simulink model "nonlinear_model1"  (R2021b)
settings: Solver=FixedStepAuto  StartTime=0.0  StopTime=RunTime  FixedStep=time_step  RelTol=1e-3
values from neighbouring files (symbols this model uses):
  g1 = (m_1 * c_1_0 + m_2 * l_1) * g    [compare_ourmodel_with_others.m]    (also in step4_0_linearize_operating_point.m = (m1 * c1 + m2 * l1) * g; step6_1_controller_feedback.m = (m1 * c1 + m2 * l1) * g)
  g2 = m_2 * c_2_0 * g    [compare_ourmodel_with_others.m]    (also in step4_0_linearize_operating_point.m = m2 * c2 * g; step6_1_controller_feedback.m = m2 * c2 * g)
  init_theta_1 = pi    (= 3.14159265359)    [compare_ourmodel_with_others.m]    (also in step2_whitebox_beam.m = theta_1(1); step2_whitebox_pend.m)
  init_theta_2 = 0    [compare_ourmodel_with_others.m]    (also in step2_whitebox_beam.m = theta_1(2); step2_whitebox_pend.m = -1.57079632679)
  P1 = m_1 * c_1_0 * c_1_0 + m_2 * l_1 * l_1 + I_1_0    [compare_ourmodel_with_others.m]    (also in step4_0_linearize_operating_point.m = m1 * c1 * c1 + m2 * l1 * l1 + I1; step6_1_controller_feedback.m = m1 * c1 * c1 + m2 * l1 * l1 + I1)
  P2 = m_2 * c_2_0 * c_2_0 + I_2_0    [compare_ourmodel_with_others.m]    (also in step4_0_linearize_operating_point.m = m2 * c2 * c2 + I2; step6_1_controller_feedback.m = m2 * c2 * c2 + I2)
  P3 = m_2 * l_1 * c_2_0    [compare_ourmodel_with_others.m]    (also in step4_0_linearize_operating_point.m = m2 * l1 * c2; step6_1_controller_feedback.m = m2 * l1 * c2)
  params = [9.81, 0.1, 0.1, 0.125, 0.0487, -0.0286, 0.0624, 0.0169, 6.81e-5, 6.9742, 2.89e-05, 46.1069, 0.0308]    [compare_ourmodel_with_others.m]    (also in costfun.m = x; step2_whitebox_pend.m = x; step4_linearized_system.mat = [9.81 0.1 0.1 0.125 0.046955 -0.032 0.04609 0.0088 9.8e-05 6)
settings Model: Creator=97083  LastModifiedBy=97083
settings DataIOCC: ExternalInput=[u]
settings DebuggingCC: UnconnectedInputMsg=none  UnconnectedOutputMsg=none  UnconnectedLineMsg=none  UnderSpecifiedDimensionMsg=warning
settings ModelReferenceCC: EnableRefExpFcnMdlSchedulingChecks=off
settings RTWCC: DLArmComputeVersion=20.02.1

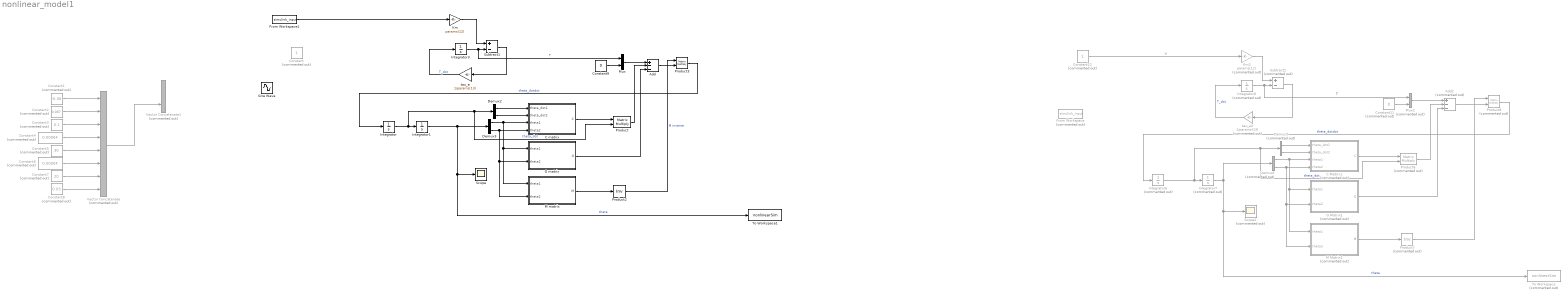
== system nonlinear_model1 ==
  Add : Sum  Inputs=+--
  Add2 : Sum  Commented=on  Inputs=+--
  C Matrix1 : MATLAB Function  Commented=on  TreatAsAtomicUnit=on
  C matrix : MATLAB Function  TreatAsAtomicUnit=on
  Constant : Constant  Commented=on
  Constant1 : Constant  Commented=on  Value=-0.06
  Constant11 : Constant  Commented=on  Value=0
  Constant12 : Constant  Commented=on
  Constant2 : Constant  Commented=on  Value=0.087
  Constant3 : Constant  Commented=on  Value=0.1
  Constant4 : Constant  Commented=on  Value=0.00004
  Constant5 : Constant  Commented=on  Value=30
  Constant6 : Constant  Commented=on  Value=0.00004
  Constant7 : Constant  Commented=on  Value=20
  Constant8 : Constant  Commented=on  Value=0.03
  Constant9 : Constant  Value=0
  Demux2 : Demux  Outputs=2
  Demux3 : Demux  Outputs=2
  Demux5 : Demux  Commented=on  Outputs=2
  Demux6 : Demux  Commented=on  Outputs=2
  From Workspace : FromWorkspace  Commented=on  SampleTime=-1
  From Workspace1 : FromWorkspace  SampleTime=-1
  G Matrix1 : MATLAB Function  Commented=on  TreatAsAtomicUnit=on
  G matrix : MATLAB Function  TreatAsAtomicUnit=on
  Integrator : Integrator
  Integrator1 : Integrator  InitialCondition=[init_theta_1, init_theta_2]
  Integrator3 : Integrator
  Integrator6 : Integrator  Commented=on
  Integrator7 : Integrator  Commented=on  InitialCondition=[init_theta_1, init_theta_2]
  Integrator8 : Integrator  Commented=on
  Km : Gain  Gain=params(12)
  Km2 : Gain  Commented=on  Gain=params(12)
  M Matrix1 : MATLAB Function  Commented=on  TreatAsAtomicUnit=on
  M matrix : MATLAB Function  TreatAsAtomicUnit=on
  Mux : Mux  Inputs=2
  Mux2 : Mux  Commented=on  Inputs=2
  Product : Product  Inputs=**  Multiplication=Matrix(*)
  Product2 : Product  Inputs=/  Multiplication=Matrix(*)
  Product3 : Product  Inputs=**  Multiplication=Matrix(*)
  Product6 : Product  Commented=on  Inputs=**  Multiplication=Matrix(*)
  Product7 : Product  Commented=on  Inputs=/  Multiplication=Matrix(*)
  Product8 : Product  Commented=on  Inputs=**  Multiplication=Matrix(*)
  Scope : Scope
  Scope2 : Scope  Commented=on
  Sine Wave : Sin  Amplitude=4  Frequency=4  SampleTime=0
  Subtract1 : Sum  Inputs=+-
  Subtract2 : Sum  Commented=on  Inputs=+-
  To Workspace : ToWorkspace  Commented=on  VariableName=nonlinearSim  SampleTime=0.001
  To Workspace1 : ToWorkspace  VariableName=nonlinearSim  SampleTime=0.001
  Vector Concatenate : Concatenate  Commented=on  NumInputs=8
  Vector Concatenate1 : Concatenate  Commented=on
  tau_e : Gain  Gain=1/params(13)
  tau_e2 : Gain  Commented=on  Gain=1/params(13)
  wires:
  Constant1/1 -> Vector Concatenate/1
  Constant2/1 -> Vector Concatenate/2
  Constant3/1 -> Vector Concatenate/3
  Constant4/1 -> Vector Concatenate/4
  Constant5/1 -> Vector Concatenate/5
  Constant6/1 -> Vector Concatenate/6
  Constant7/1 -> Vector Concatenate/7
  Constant8/1 -> Vector Concatenate/8
  ? -> Vector Concatenate1/1
  Vector Concatenate/1 -> Vector Concatenate1/2
  G matrix/1(G) -> Add/3
  From Workspace1/1 -> Km/1
  Product/1 -> Add/2
  Subtract1/1 -> tau_e/1
  Add/1 -> Product3/2
  Demux2/1 -> C matrix/1(theta_dot1)
  Constant9/1 -> Mux/2
  Integrator3/1 -> Mux/1, Subtract1/2  "T"
  tau_e/1 -> Integrator3/1  "T_dot"
  Demux3/1 -> M matrix/1(theta1), G matrix/1(theta1), C matrix/3(theta1)
  Product2/1 -> Product3/1  "M inverse"
  Product3/1 -> Integrator/1  "theta_dotdot"
  Km/1 -> Subtract1/1
  Demux3/2 -> M matrix/2(theta2), G matrix/2(theta2), C matrix/4(theta2)
  M matrix/1(M) -> Product2/1
  Demux2/2 -> C matrix/2(theta_dot2)
  Integrator1/1 -> Demux3/1, To Workspace1/1, Scope/1  "theta"
  Mux/1 -> Add/1
  C matrix/1(C) -> Product/1
  Integrator/1 -> Product/2, Demux2/1, Integrator1/1  "theta_dot"
  Constant12/1 -> Km2/1  "u"
  Product7/1 -> Product8/1
  Demux6/1 -> M Matrix1/1(theta1), G Matrix1/1(theta1), C Matrix1/3(theta1)
  Demux6/2 -> M Matrix1/2(theta2), G Matrix1/2(theta2), C Matrix1/4(theta2)
  Integrator6/1 -> Product6/2, Demux5/1, Integrator7/1  "theta_dot"
  Add2/1 -> Product8/2
  Demux5/1 -> C Matrix1/1(theta_dot1)
  Mux2/1 -> Add2/1
  Km2/1 -> Subtract2/1
  Constant11/1 -> Mux2/2
  Product6/1 -> Add2/2
  Integrator8/1 -> Mux2/1, Subtract2/2  "T"
  Integrator7/1 -> To Workspace/1, Scope2/1, Demux6/1  "theta"
  Subtract2/1 -> tau_e2/1
  Product8/1 -> Integrator6/1  "theta_dotdot"
  tau_e2/1 -> Integrator8/1  "T_dot"
  C Matrix1/1(C) -> Product6/1
  M Matrix1/1(M) -> Product7/1
  Demux5/2 -> C Matrix1/2(theta_dot2)
  G Matrix1/1(G) -> Add2/3

== matlab function nonlinear_model1/C matrix ==
  data: theta_dot1 input; theta_dot2 input; theta1 input; theta2 input; C output; params parameter; P3 parameter
function C = C(theta_dot1, theta_dot2, theta1, theta2, params, P3)
C00 = params(10) - P3 * theta_dot2 * sin(theta2);
C01 = -P3 * (theta_dot1 + theta_dot2) * sin(theta2);
C10 = P3 * theta_dot1 * sin(theta2);
C11 = params(11);

C = [C00 C01; C10 C11];

== matlab function nonlinear_model1/G matrix ==
  data: theta1 input; theta2 input; G output; g1 parameter; g2 parameter
function G = G(theta1, theta2, g1, g2)
G00 = -g1 * sin(theta1) - g2 * sin(theta1 + theta2);
G01 = -g2 * sin(theta1 + theta2);

G = [G00 G01];

== matlab function nonlinear_model1/M matrix ==
  data: theta1 input; theta2 input; M output; P1 parameter; P2 parameter; P3 parameter
function M = M(theta1, theta2, P1, P2, P3)
M00 = P1 + P2 + 2 * P3 * cos(theta2);
M01 = P2 + P3 * cos(theta2);
M10 = M01;
M11 = P2;

M = [M00 M01; M10 M11];

== matlab function nonlinear_model1/C Matrix1 ==
  data: theta_dot1 input; theta_dot2 input; theta1 input; theta2 input; C output; params parameter; P3 parameter
function C = C(theta_dot1, theta_dot2, theta1, theta2, params, P3)
C00 = params(10)-P3*theta_dot2*sin(theta2);
C01 = -P3*(theta_dot1+theta_dot2)*sin(theta2);
C10 = P3*theta_dot1*sin(theta2);
C11 = params(11);
C = [C00 C01; C10 C11];

== matlab function nonlinear_model1/G Matrix1 ==
  data: theta1 input; theta2 input; G output; g1 parameter; g2 parameter
function G = G(theta1, theta2, g1, g2)
g00 = -g1*sin(theta1)-g2*sin(theta1+theta2);
g01 = -g2*sin(theta1+theta2);
G = [g00 g01];

== matlab function nonlinear_model1/M Matrix1 ==
  data: theta1 input; theta2 input; M output; P1 parameter; P2 parameter; P3 parameter
function M = M(theta1, theta2, P1, P2, P3)
m00 = P1+P2+2*P3*cos(theta2);
m01 = P2+P3*cos(theta2);
m10 = m01;
m11 = P2;
M = [m00 m01; m10 m11];
